simulink model "CULARIS_Aero"  (Simulink 8.2)
settings: Solver=ode45  StartTime=0.0  StopTime=10.0  RelTol=1e-3
undefined symbols (not defined in the file or in its folder): uavsim
libraries: aerolibadyn x1, uavsimBlockset_DerivedAerodynamicConditions x1
settings Model: Creator=mstolle  LastModifiedBy=mstolle
settings DataIOCC: SignalLoggingSaveFormat=Dataset
settings OptimizationCC: ExpressionDepthLimit=128
settings DebuggingCC: FcnCallInpInsideContextMsg=EnableAllAsError  StateNameClashWarn=none
settings GRTTargetCC: CombineOutputUpdateFcns=on  GRTInterface=off

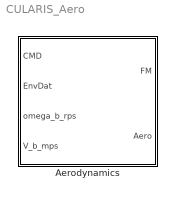
== system CULARIS_Aero ==
  Aerodynamics : Subsystem

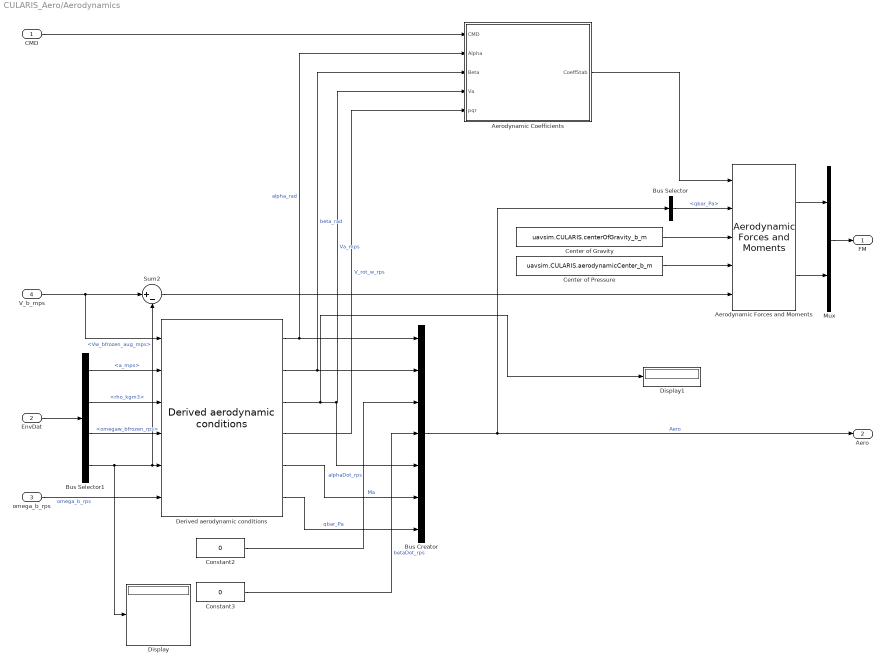
== system CULARIS_Aero/Aerodynamics ==
  CMD : Inport  OutDataTypeStr=Bus: CMD
  EnvDat : Inport  Port=2  OutDataTypeStr=Bus: EnvironmentAug
  omega_b_rps : Inport  Port=3
  V_b_mps : Inport  Port=4
  Aerodynamic Coefficients : Subsystem
  "Aerodynamic Forces and Moments " : aerolibadyn/Aerodynamic Forces and Moments   inputAxes=Wind  outputForceAxes=Body  outputMomentAxes=Body  S=uavsim.CULARIS.S  b=uavsim.CULARIS.b  cbar=uavsim.CULARIS.c
  Bus Creator : BusCreator  Inputs=7  OutDataTypeStr=Bus: Aero  NonVirtualBus=on
  Bus Selector1 : BusSelector  OutputSignals=Environment.a_mps,Environment.rho_kgm3,Environment.omegaw_bfrozen_rps,Vw_bfrozen_aug_mps
  Bus Selector : BusSelector  OutputSignals=qbar_Pa
  Center of Gravity : Constant  Value=uavsim.CULARIS.centerOfGravity_b_m  SampleTime=0
  Center of Pressure : Constant  Value=uavsim.CULARIS.aerodynamicCenter_b_m  SampleTime=0
  Constant2 : Constant  Value=0
  Constant3 : Constant  Value=0
  Derived aerodynamic conditions : uavsimBlockset_DerivedAerodynamicConditions/Derived aerodynamic conditions
  Display : Display
  Display1 : Display
  Mux : Mux  Inputs=2
  Sum2 : Sum  Inputs=|+-  SaturateOnIntegerOverflow=on  InputSameDT=on  OutDataTypeStr=Inherit: Same as first input
  FM : Outport
  Aero : Outport  Port=2
  wires:
  Derived aerodynamic conditions/6 -> Bus Creator/7  "qbar_Pa"
  Constant3/1 -> Bus Creator/4  "betaDot_rps"
  Constant2/1 -> Bus Creator/3  "alphaDot_rps"
  Derived aerodynamic conditions/5 -> Bus Creator/6  "Ma"
  Derived aerodynamic conditions/4 -> Aerodynamic Coefficients/5(pqr)  "V_rot_w_rps"
  omega_b_rps/1 -> Derived aerodynamic conditions/6  "omega_b_rps"
  Bus Selector1/4 -> Display/1, Derived aerodynamic conditions/5, Sum2/2  "<Vw_bfrozen_aug_mps>"
  Bus Selector1/3 -> Derived aerodynamic conditions/4  "<omegaw_bfrozen_rps>"
  Bus Selector1/2 -> Derived aerodynamic conditions/3  "<rho_kgm3>"
  Bus Selector/1 -> "Aerodynamic Forces and Moments "/2  "<qbar_Pa>"
  Mux/1 -> FM/1
  EnvDat/1 -> Bus Selector1/1
  Derived aerodynamic conditions/1 -> Bus Creator/1, Aerodynamic Coefficients/2(Alpha)  "alpha_rad"
  Derived aerodynamic conditions/2 -> Bus Creator/2, Aerodynamic Coefficients/3(Beta)  "beta_rad"
  CMD/1 -> Aerodynamic Coefficients/1(CMD)
  Derived aerodynamic conditions/3 -> Aerodynamic Coefficients/4(Va), Bus Creator/5, Display1/1  "Va_mps"
  Center of Pressure/1 -> "Aerodynamic Forces and Moments "/4
  Center of Gravity/1 -> "Aerodynamic Forces and Moments "/3
  "Aerodynamic Forces and Moments "/1 -> Mux/1
  Bus Selector1/1 -> Derived aerodynamic conditions/2  "<a_mps>"
  Bus Creator/1 -> Aero/1, Bus Selector/1  "Aero"
  Aerodynamic Coefficients/1(CoeffStab) -> "Aerodynamic Forces and Moments "/1
  "Aerodynamic Forces and Moments "/2 -> Mux/2
  Sum2/1 -> "Aerodynamic Forces and Moments "/5
  V_b_mps/1 -> Sum2/1, Derived aerodynamic conditions/1

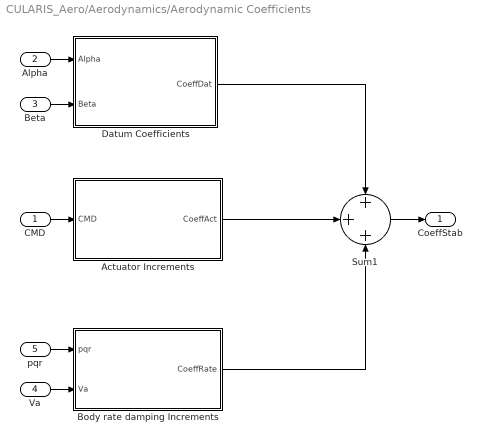
== system CULARIS_Aero/Aerodynamics/Aerodynamic Coefficients ==
  CMD : Inport
  Alpha : Inport  Port=2
  Beta : Inport  Port=3
  Va : Inport  Port=4
  pqr : Inport  Port=5
  Actuator Increments : Subsystem
  Body rate damping Increments : Subsystem
  Datum Coefficients : Subsystem
  Sum1 : Sum  Inputs=+++  SaturateOnIntegerOverflow=on  InputSameDT=on  OutDataTypeStr=Inherit: Same as first input
  CoeffStab : Outport
  wires:
  Datum Coefficients/1(CoeffDat) -> Sum1/1
  Sum1/1 -> CoeffStab/1
  CMD/1 -> Actuator Increments/1(CMD)
  Beta/1 -> Datum Coefficients/2(Beta)
  pqr/1 -> Body rate damping Increments/1(pqr)
  Va/1 -> Body rate damping Increments/2(Va)
  Alpha/1 -> Datum Coefficients/1(Alpha)
  Body rate damping Increments/1(CoeffRate) -> Sum1/3
  Actuator Increments/1(CoeffAct) -> Sum1/2

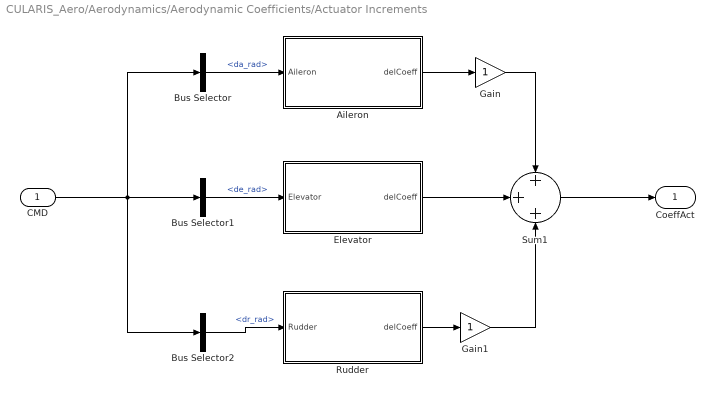
== system CULARIS_Aero/Aerodynamics/Aerodynamic Coefficients/Actuator Increments ==
  CMD : Inport
  Aileron : Subsystem
  Bus Selector : BusSelector  OutputSignals=da_rad
  Bus Selector1 : BusSelector  OutputSignals=de_rad
  Bus Selector2 : BusSelector  OutputSignals=dr_rad
  Elevator : Subsystem
  Gain : Gain
  Gain1 : Gain
  Rudder : Subsystem
  Sum1 : Sum  Inputs=+++  SaturateOnIntegerOverflow=on  InputSameDT=on  OutDataTypeStr=Inherit: Same as first input
  CoeffAct : Outport  InitialOutput=0
  wires:
  Elevator/1(delCoeff) -> Sum1/2
  Aileron/1(delCoeff) -> Gain/1
  Rudder/1(delCoeff) -> Gain1/1
  Sum1/1 -> CoeffAct/1
  CMD/1 -> Bus Selector/1, Bus Selector1/1, Bus Selector2/1
  Bus Selector2/1 -> Rudder/1(Rudder)  "<dr_rad>"
  Bus Selector1/1 -> Elevator/1(Elevator)  "<de_rad>"
  Bus Selector/1 -> Aileron/1(Aileron)  "<da_rad>"
  Gain/1 -> Sum1/1
  Gain1/1 -> Sum1/3

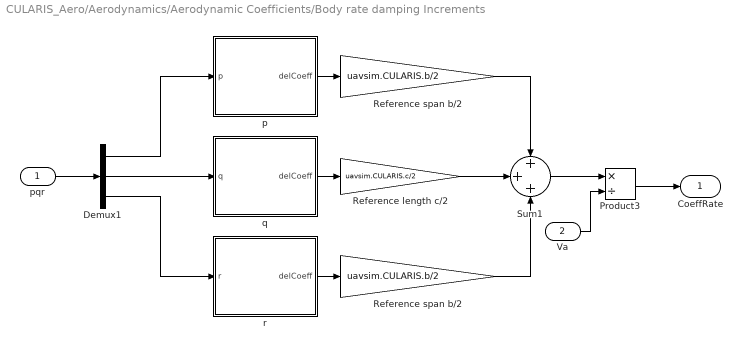
== system CULARIS_Aero/Aerodynamics/Aerodynamic Coefficients/Body rate damping Increments ==
  pqr : Inport
  Va : Inport  Port=2
  Demux1 : Demux  Outputs=3
  Product3 : Product  Inputs=*/  SaturateOnIntegerOverflow=on  InputSameDT=on  OutDataTypeStr=Inherit: Same as first input
  Reference length c/2 : Gain  Gain=uavsim.CULARIS.c/2
  Reference span b/2 : Gain  Gain=uavsim.CULARIS.b/2
  "Reference span b/2 " : Gain  Gain=uavsim.CULARIS.b/2
  Sum1 : Sum  Inputs=+++  SaturateOnIntegerOverflow=on  InputSameDT=on  OutDataTypeStr=Inherit: Same as first input
  p : Subsystem
  q : Subsystem
  r : Subsystem
  CoeffRate : Outport  InitialOutput=0
  wires:
  "Reference span b/2 "/1 -> Sum1/1
  Reference length c/2/1 -> Sum1/2
  Reference span b/2/1 -> Sum1/3
  Va/1 -> Product3/2
  Sum1/1 -> Product3/1
  Product3/1 -> CoeffRate/1
  r/1(delCoeff) -> Reference span b/2/1
  q/1(delCoeff) -> Reference length c/2/1
  p/1(delCoeff) -> "Reference span b/2 "/1
  Demux1/3 -> r/1(r)
  Demux1/2 -> q/1(q)
  Demux1/1 -> p/1(p)
  pqr/1 -> Demux1/1

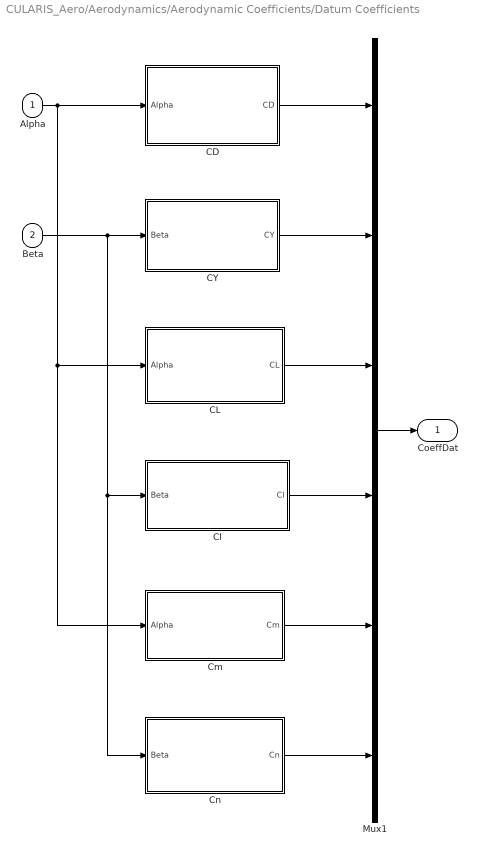
== system CULARIS_Aero/Aerodynamics/Aerodynamic Coefficients/Datum Coefficients ==
  Alpha : Inport
  Beta : Inport  Port=2
  CD : Subsystem
  CL : Subsystem
  CY : Subsystem
  Cl : Subsystem
  Cm : Subsystem
  Cn : Subsystem
  Mux1 : Mux  Inputs=6
  CoeffDat : Outport  InitialOutput=0
  wires:
  CL/1(CL) -> Mux1/3
  CD/1(CD) -> Mux1/1
  CY/1(CY) -> Mux1/2
  Cl/1("Cl ") -> Mux1/4
  Cm/1(Cm) -> Mux1/5
  Cn/1(Cn) -> Mux1/6
  Beta/1 -> CY/1("Beta "), Cl/1(Beta), Cn/1(Beta)
  Alpha/1 -> Cm/1(Alpha), CL/1(Alpha), CD/1(Alpha)
  Mux1/1 -> CoeffDat/1

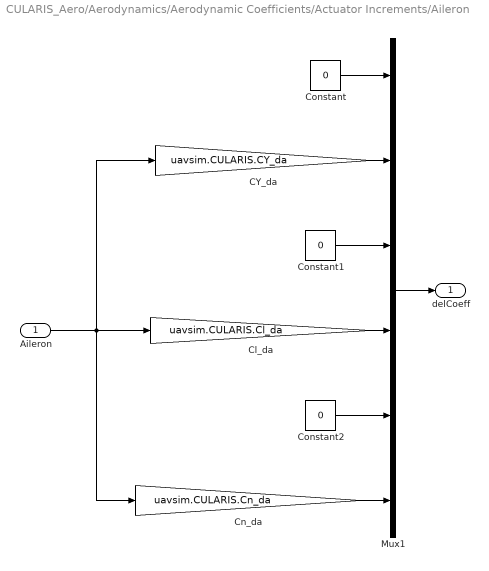
== system CULARIS_Aero/Aerodynamics/Aerodynamic Coefficients/Actuator Increments/Aileron ==
  Aileron : Inport
  CY_da : Gain  Gain=uavsim.CULARIS.CY_da
  Cl_da : Gain  Gain=uavsim.CULARIS.Cl_da
  Cn_da : Gain  Gain=uavsim.CULARIS.Cn_da
  Constant : Constant  Value=0
  Constant1 : Constant  Value=0
  Constant2 : Constant  Value=0
  Mux1 : Mux  Inputs=6
  delCoeff : Outport
  wires:
  Cn_da/1 -> Mux1/6
  Cl_da/1 -> Mux1/4
  CY_da/1 -> Mux1/2
  Mux1/1 -> delCoeff/1
  Constant/1 -> Mux1/1
  Aileron/1 -> CY_da/1, Cn_da/1, Cl_da/1
  Constant1/1 -> Mux1/3
  Constant2/1 -> Mux1/5

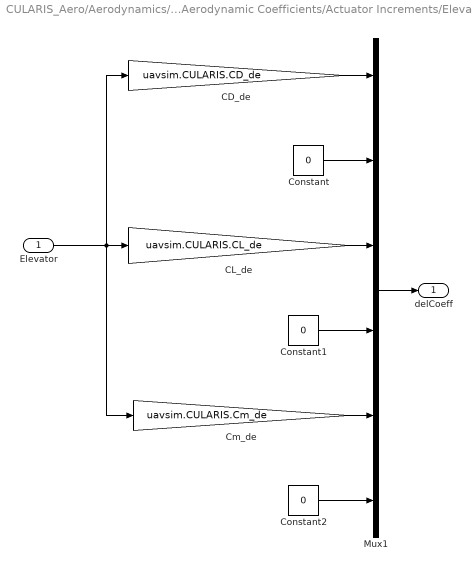
== system CULARIS_Aero/Aerodynamics/Aerodynamic Coefficients/Actuator Increments/Elevator ==
  Elevator : Inport
  CD_de : Gain  Gain=uavsim.CULARIS.CD_de
  CL_de : Gain  Gain=uavsim.CULARIS.CL_de
  Cm_de : Gain  Gain=uavsim.CULARIS.Cm_de
  Constant : Constant  Value=0
  Constant1 : Constant  Value=0
  Constant2 : Constant  Value=0
  Mux1 : Mux  Inputs=6
  delCoeff : Outport
  wires:
  Constant/1 -> Mux1/2
  Cm_de/1 -> Mux1/5
  CL_de/1 -> Mux1/3
  Mux1/1 -> delCoeff/1
  CD_de/1 -> Mux1/1
  Elevator/1 -> Cm_de/1, CD_de/1, CL_de/1
  Constant1/1 -> Mux1/4
  Constant2/1 -> Mux1/6

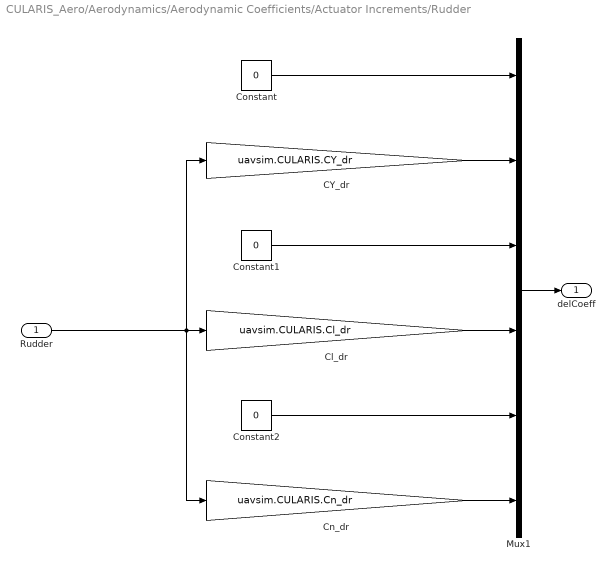
== system CULARIS_Aero/Aerodynamics/Aerodynamic Coefficients/Actuator Increments/Rudder ==
  Rudder : Inport
  CY_dr : Gain  Gain=uavsim.CULARIS.CY_dr
  Cl_dr : Gain  Gain=uavsim.CULARIS.Cl_dr
  Cn_dr : Gain  Gain=uavsim.CULARIS.Cn_dr
  Constant : Constant  Value=0
  Constant1 : Constant  Value=0
  Constant2 : Constant  Value=0
  Mux1 : Mux  Inputs=6
  delCoeff : Outport
  wires:
  Constant/1 -> Mux1/1
  Cn_dr/1 -> Mux1/6
  Cl_dr/1 -> Mux1/4
  CY_dr/1 -> Mux1/2
  Mux1/1 -> delCoeff/1
  Rudder/1 -> CY_dr/1, Cn_dr/1, Cl_dr/1
  Constant1/1 -> Mux1/3
  Constant2/1 -> Mux1/5

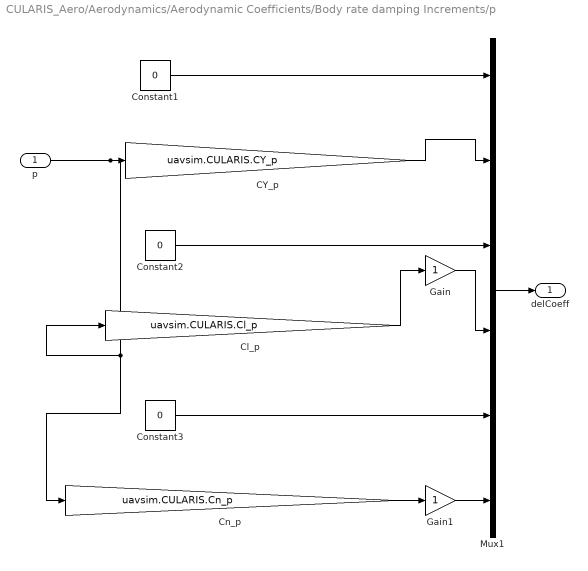
== system CULARIS_Aero/Aerodynamics/Aerodynamic Coefficients/Body rate damping Increments/p ==
  p : Inport
  CY_p : Gain  Gain=uavsim.CULARIS.CY_p
  Cl_p : Gain  Gain=uavsim.CULARIS.Cl_p
  Cn_p : Gain  Gain=uavsim.CULARIS.Cn_p
  Constant1 : Constant  Value=0
  Constant2 : Constant  Value=0
  Constant3 : Constant  Value=0
  Gain : Gain
  Gain1 : Gain
  Mux1 : Mux  Inputs=6
  delCoeff : Outport
  wires:
  p/1 -> Cn_p/1, Cl_p/1, CY_p/1
  CY_p/1 -> Mux1/2
  Constant1/1 -> Mux1/1
  Cn_p/1 -> Gain1/1
  Cl_p/1 -> Gain/1
  Mux1/1 -> delCoeff/1
  Constant2/1 -> Mux1/3
  Constant3/1 -> Mux1/5
  Gain/1 -> Mux1/4
  Gain1/1 -> Mux1/6

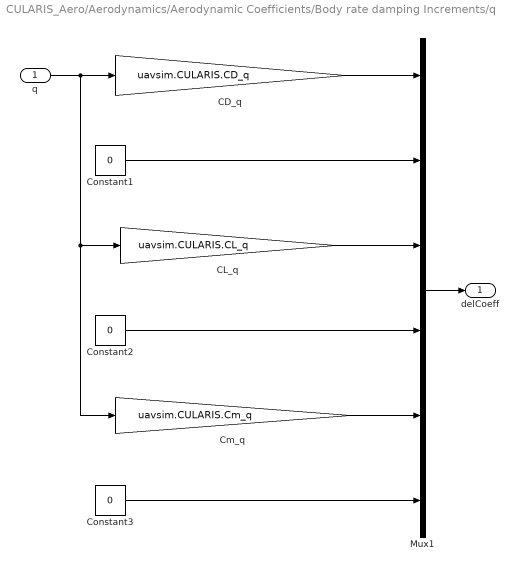
== system CULARIS_Aero/Aerodynamics/Aerodynamic Coefficients/Body rate damping Increments/q ==
  q : Inport
  CD_q : Gain  Gain=uavsim.CULARIS.CD_q
  CL_q : Gain  Gain=uavsim.CULARIS.CL_q
  Cm_q : Gain  Gain=uavsim.CULARIS.Cm_q
  Constant1 : Constant  Value=0
  Constant2 : Constant  Value=0
  Constant3 : Constant  Value=0
  Mux1 : Mux  Inputs=6
  delCoeff : Outport
  wires:
  Cm_q/1 -> Mux1/5
  CL_q/1 -> Mux1/3
  CD_q/1 -> Mux1/1
  Constant1/1 -> Mux1/2
  q/1 -> Cm_q/1, CL_q/1, CD_q/1
  Mux1/1 -> delCoeff/1
  Constant2/1 -> Mux1/4
  Constant3/1 -> Mux1/6

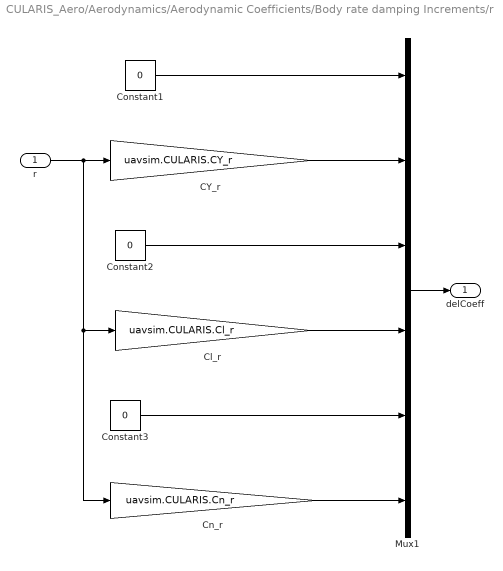
== system CULARIS_Aero/Aerodynamics/Aerodynamic Coefficients/Body rate damping Increments/r ==
  r : Inport
  CY_r : Gain  Gain=uavsim.CULARIS.CY_r
  Cl_r : Gain  Gain=uavsim.CULARIS.Cl_r
  Cn_r : Gain  Gain=uavsim.CULARIS.Cn_r
  Constant1 : Constant  Value=0
  Constant2 : Constant  Value=0
  Constant3 : Constant  Value=0
  Mux1 : Mux  Inputs=6
  delCoeff : Outport
  wires:
  Cn_r/1 -> Mux1/6
  Cl_r/1 -> Mux1/4
  CY_r/1 -> Mux1/2
  Constant1/1 -> Mux1/1
  r/1 -> Cn_r/1, Cl_r/1, CY_r/1
  Mux1/1 -> delCoeff/1
  Constant2/1 -> Mux1/3
  Constant3/1 -> Mux1/5

== system CULARIS_Aero/Aerodynamics/Aerodynamic Coefficients/Datum Coefficients/CD ==
  Alpha : Inport
  CD_0 : Constant  Value=uavsim.CULARIS.CD_0
  CL_0 : Constant  Value=uavsim.CULARIS.CL_0
  CL_alpha : Gain  Gain=uavsim.CULARIS.CL_alpha
  Product : Product  RndMeth=Zero
  Sum1 : Sum  Inputs=|++
  Sum2 : Sum  Inputs=|++
  sec. order lift contribution : Gain  Gain=1/(pi*uavsim.CULARIS.oswald*uavsim.CULARIS.AR )
  CD : Outport
  wires:
  CL_alpha/1 -> Sum2/2
  Alpha/1 -> CL_alpha/1
  Sum1/1 -> CD/1
  CD_0/1 -> Sum1/2
  sec. order lift contribution/1 -> Sum1/1
  Product/1 -> sec. order lift contribution/1
  Sum2/1 -> Product/1, Product/2
  CL_0/1 -> Sum2/1

== system CULARIS_Aero/Aerodynamics/Aerodynamic Coefficients/Datum Coefficients/CL ==
  note: CL_0
  Alpha : Inport
  1 : Constant  Value=uavsim.CULARIS.CL_0
  CL_alpha : Gain  Gain=uavsim.CULARIS.CL_alpha
  Sum2 : Sum  Inputs=|++
  CL : Outport
  wires:
  Sum2/1 -> CL/1
  CL_alpha/1 -> Sum2/1
  Alpha/1 -> CL_alpha/1
  1/1 -> Sum2/2

== system CULARIS_Aero/Aerodynamics/Aerodynamic Coefficients/Datum Coefficients/CY ==
  "Beta " : Inport
  "CY_0 " : Constant  Value=uavsim.CULARIS.CY_0
  CY_beta : Gain  Gain=uavsim.CULARIS.CY_beta  SaturateOnIntegerOverflow=on  OutDataTypeStr=Inherit: Same as input  ParamDataTypeStr=Inherit: Same as input
  Sum : Sum  Inputs=|++
  CY : Outport
  wires:
  "CY_0 "/1 -> Sum/1
  CY_beta/1 -> Sum/2
  Sum/1 -> CY/1
  "Beta "/1 -> CY_beta/1

== system CULARIS_Aero/Aerodynamics/Aerodynamic Coefficients/Datum Coefficients/Cl ==
  Beta : Inport
  "Cl_0 " : Constant  Value=uavsim.CULARIS.Cl_0
  Cl_beta : Gain  Gain=uavsim.CULARIS.Cl_beta  SaturateOnIntegerOverflow=on  OutDataTypeStr=Inherit: Same as input  ParamDataTypeStr=Inherit: Same as input
  Sum1 : Sum  Inputs=|++
  "Cl " : Outport
  wires:
  Beta/1 -> Cl_beta/1
  Sum1/1 -> "Cl "/1
  "Cl_0 "/1 -> Sum1/2
  Cl_beta/1 -> Sum1/1

== system CULARIS_Aero/Aerodynamics/Aerodynamic Coefficients/Datum Coefficients/Cm ==
  Alpha : Inport
  Cm_0 : Constant  Value=uavsim.CULARIS.Cm_0
  Cm_alpha : Gain  Gain=uavsim.CULARIS.Cm_alpha  SaturateOnIntegerOverflow=on  OutDataTypeStr=Inherit: Same as input  ParamDataTypeStr=Inherit: Same as input
  Sum2 : Sum  Inputs=|++
  Cm : Outport
  wires:
  Alpha/1 -> Cm_alpha/1
  Cm_alpha/1 -> Sum2/1
  Sum2/1 -> Cm/1
  Cm_0/1 -> Sum2/2

== system CULARIS_Aero/Aerodynamics/Aerodynamic Coefficients/Datum Coefficients/Cn ==
  Beta : Inport
  Cn_0 : Constant  Value=uavsim.CULARIS.Cn_0
  Cn_beta : Gain  Gain=uavsim.CULARIS.Cn_beta  SaturateOnIntegerOverflow=on  OutDataTypeStr=Inherit: Same as input  ParamDataTypeStr=Inherit: Same as input
  Sum3 : Sum  Inputs=|++
  Cn : Outport
  wires:
  Beta/1 -> Cn_beta/1
  Cn_beta/1 -> Sum3/1
  Sum3/1 -> Cn/1
  Cn_0/1 -> Sum3/2
